simulink model "BaseEngineController_LS_128"  (Simulink 7.7)
settings: Solver=FixedStepDiscrete  StartTime=0.0  StopTime=10.0  RelTol=1e-3
PreLoadFcn:
  | try, eval([bdroot '_setup']); catch, eval('model_setup', ''); end
InitFcn:
  | try, eval([bdroot '_setup']); catch, eval('model_setup', ''); end
undefined symbols (not defined in the file): ECU565, High, motohawk_build_version, motohawk_trunc_name, motohawk_vardec_config_group, motohawk_vardec_path, True
libraries: MotoHawk_lib x1418, motohawk_control_primitives_lib x183, motohawk_engine_lib x32, simulink x21, motohawk_annotations_lib x9, AutoDoc_lib x8, simulink_extras x4, motohawk_ccp_examples_lib x1, motohawk_control_primitives_motoshare_lib x1
(part 25 of 27)

== system BaseEngineController_LS_128/Foreground/Control/Controller/Run/Fuel System Manager/O2 Fuel Adapt/Saturation (Tunable)1 ==
  note: Calibratable wrapper around the Saturation block
  In : Inport
  Saturation : motohawk_control_primitives_lib/Saturation  SystemSampleTime=-1
  motohawk_calibration : MotoHawk_lib/Calibration & Probing Blocks/motohawk_calibration  nam=[prefix 'LwrLim']  val=LwrLim  storage=Calibration  show_more=on  name_source=Use Parameter  data_type=Inherit via back propagation  read_level=1  write_level=1  ovr_cals=on  view_as=Number  enum_struct={'Disabled', 'Enabled'}  vector_style=Wide Row  use_help_units=off  help='Lower Limit Value'  units=units  use_header_enum=off  row_header_enum={}  col_header_enum={}  use_min_max=on  min_val=-inf  max_val=inf  use_precision=on  precision='1.4'  gain=1  offset=0  exp=1  use_mototune_group=on  mototune_group=motohawk_vardec_path(gcb)
  motohawk_calibration1 : MotoHawk_lib/Calibration & Probing Blocks/motohawk_calibration  nam=[prefix 'UprLim']  val=UprLim  storage=Calibration  show_more=on  name_source=Use Parameter  data_type=Inherit via back propagation  read_level=1  write_level=1  ovr_cals=on  view_as=Number  enum_struct={'Disabled', 'Enabled'}  vector_style=Wide Row  use_help_units=off  help='Upper Limit Value'  units=units  use_header_enum=off  row_header_enum={}  col_header_enum={}  use_min_max=on  min_val=-inf  max_val=inf  use_precision=on  precision='1.4'  gain=1  offset=0  exp=1  use_mototune_group=on  mototune_group=motohawk_vardec_path(gcb)
  Out : Outport
  wires:
  motohawk_calibration1/1 -> Saturation/3
  In/1 -> Saturation/1
  motohawk_calibration/1 -> Saturation/2
  Saturation/1 -> Out/1

== system BaseEngineController_LS_128/Foreground/Control/Controller/Run/Fuel System Manager/O2 Fuel Adapt/WarmUp Disable ==
  WarmupRatio : Inport
  WarmupTimeRatio : Inport  Port=2
  BaseRatio : Inport  Port=3
  Constant : Constant  Value=0.01
  Logical Operator : Logic  Operator=NOT  AllPortsSameDT=off
  MinMax : MinMax  Function=max  Inputs=2
  Relational Operator : RelationalOperator  Operator=>  InputSameDT=on
  Sum : Sum  Inputs=|+-
  motohawk_probe5 : MotoHawk_lib/Calibration & Probing Blocks/motohawk_probe  nam='WarmUpO2AdaptEnabled'  show_more=on  name_source=Use Parameter  read_level=1  view_as=Enumeration  enum_struct={'Not Enabled', 'Enabled'}  vector_style=Wide Row  use_help_units=on  help='Indicates whether FuelFlowComp map adapting is enabled due to WarmUp'  units=''  use_header_enum=off  row_header_enum={}  col_header_enum={}  use_precision=off  precision=''  gain=1  offset=0  exp=1  use_mototune_group=on  mototune_group=motohawk_vardec_path(gcb)
  State_Out : Outport
  wires:
  Relational Operator/1 -> Logical Operator/1
  Logical Operator/1 -> State_Out/1, motohawk_probe5/1
  Constant/1 -> Relational Operator/2
  WarmupRatio/1 -> MinMax/1
  WarmupTimeRatio/1 -> MinMax/2
  MinMax/1 -> Sum/1
  BaseRatio/1 -> Sum/2
  Sum/1 -> Relational Operator/1

== system BaseEngineController_LS_128/Foreground/Control/Controller/Run/MaxGovernor/Trigger Pre-load/InGear ==
  Enable : EnablePort
  Saturation : motohawk_control_primitives_lib/Saturation  SystemSampleTime=-1
  motohawk_calibration2 : MotoHawk_lib/Calibration & Probing Blocks/motohawk_calibration  nam='MaxGovInGearRPMSetPt'  val=4200  storage=Calibration  show_more=on  name_source=Use Parameter  data_type=uint16  read_level=1  write_level=1  ovr_cals=on  view_as=Number  enum_struct={'Disabled', 'Enabled'}  vector_style=Wide Row  use_help_units=on  help='Max Gov RPM setpoint when in gear.'  units='RPM'  use_header_enum=off  row_header_enum={}  col_header_enum={}  use_min_max=on  min_val=0  max_val=inf  use_precision=off  precision=''  gain=1  offset=0  exp=1  use_mototune_group=on  mototune_group=motohawk_vardec_path(gcb)
  motohawk_calibration3 : MotoHawk_lib/Calibration & Probing Blocks/motohawk_calibration  nam='MaxGovInGearLowerLim'  val=300  storage=Calibration  show_more=on  name_source=Use Parameter  data_type=uint16  read_level=1  write_level=1  ovr_cals=on  view_as=Number  enum_struct={'Disabled', 'Enabled'}  vector_style=Wide Row  use_help_units=on  help='Max Gov RPM setpoint when in gear.'  units='RPM'  use_header_enum=off  row_header_enum={}  col_header_enum={}  use_min_max=on  min_val=0  max_val=inf  use_precision=off  precision=''  gain=1  offset=0  exp=1  use_mototune_group=on  mototune_group=motohawk_vardec_path(gcb)
  motohawk_calibration4 : MotoHawk_lib/Calibration & Probing Blocks/motohawk_calibration  nam='MaxGovInGearRPMThresh'  val=300  storage=Calibration  show_more=on  name_source=Use Parameter  data_type=uint16  read_level=1  write_level=1  ovr_cals=on  view_as=Number  enum_struct={'Disabled', 'Enabled'}  vector_style=Wide Row  use_help_units=on  help='When in-gear, RPM has to pass the base RPM setpoint minus this calibration. to start the I term preload and ramp-in.'  units='RPM'  use_header_enum=off  row_header_enum={}  col_header_enum={}  use_min_max=off  min_val=0  max_val=inf  use_precision=off  precision=''  gain=1  offset=0  exp=1  use_mototune_group=on  mototune_group=motohawk_vardec_path(gcb)
  motohawk_calibration5 : MotoHawk_lib/Calibration & Probing Blocks/motohawk_calibration  nam='MaxGovInGearUpperLim'  val=4200  storage=Calibration  show_more=on  name_source=Use Parameter  data_type=uint16  read_level=1  write_level=1  ovr_cals=on  view_as=Number  enum_struct={'Disabled', 'Enabled'}  vector_style=Wide Row  use_help_units=on  help='Max Gov RPM setpoint when in gear.'  units='RPM'  use_header_enum=off  row_header_enum={}  col_header_enum={}  use_min_max=on  min_val=0  max_val=inf  use_precision=off  precision=''  gain=1  offset=0  exp=1  use_mototune_group=on  mototune_group=motohawk_vardec_path(gcb)
  motohawk_data_def : MotoHawk_lib/Data Storage Blocks/motohawk_data_def  nam='MaxGovInGearSetPoint'  container_nam=''  data=3500  typ=uint16  struct_nam='MyStruct'  storage=NonVolatile  outputRef=off  use_vardec=off  window=Calibration  read_level=1  write_level=1  ovr_cals=on  view_as=Number  enum_struct={'Disabled', 'Enabled'}  vector_style=Wide Row  use_help_units=on  help=''  units=''  use_header_enum=off  row_header_enum=''  col_header_enum=''  use_min_max=off  min_val=-inf  max_val=inf  use_precision=off  precision=''  gain=1  offset=0  exp=1  use_mototune_group=off  mototune_group=motohawk_vardec_path(gcb)  eval_name=MaxGovInGearSetPoint  data_stores=motohawk_sfun_data_def_data_stores  struct_instances=motohawk_sfun_data_def_struct_instances  vardecs=motohawk_sfun_data_def_vardecs
  motohawk_data_read : MotoHawk_lib/Data Storage Blocks/motohawk_data_read  source=Lookup By Name  structure=Scalar  operation=Read scalar from location by index  sz_vec=4  sz_row=2  sz_col=3  typ=uint16  nam='MaxGovInGearSetPoint'  checkNull=on  struct_inst_name='Struct1'  struct_nam='MyStruct'
  motohawk_data_write1 : MotoHawk_lib/Data Storage Blocks/motohawk_data_write  source=Lookup By Name  structure=Scalar  operation=Write scalar into location by index  sz_vec=-1  sz_row=3  sz_col=2  typ=uint16  nam='MaxGovInGearSetPoint'  checkNull=on  write_read_only=off  struct_inst_name='Struct1'  struct_name='MyStruct'
  BaseSetpoint : Outport
  Threshold : Outport  Port=2
  wires:
  motohawk_calibration4/1 -> Threshold/1
  motohawk_calibration2/1 -> motohawk_data_write1/1
  motohawk_data_read/1 -> Saturation/1
  Saturation/1 -> BaseSetpoint/1
  motohawk_calibration3/1 -> Saturation/2
  motohawk_calibration5/1 -> Saturation/3

== system BaseEngineController_LS_128/Foreground/Control/Controller/Run/MaxGovernor/Trigger Pre-load/InNeutral ==
  Enable : EnablePort
  Saturation : motohawk_control_primitives_lib/Saturation  SystemSampleTime=-1
  motohawk_calibration2 : MotoHawk_lib/Calibration & Probing Blocks/motohawk_calibration  nam='MaxGovNtrlLowerLim'  val=2000  storage=Calibration  show_more=on  name_source=Use Parameter  data_type=uint16  read_level=1  write_level=1  ovr_cals=on  view_as=Number  enum_struct={'Disabled', 'Enabled'}  vector_style=Wide Row  use_help_units=on  help='Max Gov RPM setpoint when in gear.'  units='RPM'  use_header_enum=off  row_header_enum={}  col_header_enum={}  use_min_max=on  min_val=0  max_val=inf  use_precision=off  precision=''  gain=1  offset=0  exp=1  use_mototune_group=on  mototune_group=motohawk_vardec_path(gcb)
  motohawk_calibration3 : MotoHawk_lib/Calibration & Probing Blocks/motohawk_calibration  nam='MaxGovNtrlRPMThresh'  val=300  storage=Calibration  show_more=on  name_source=Use Parameter  data_type=uint16  read_level=1  write_level=1  ovr_cals=on  view_as=Number  enum_struct={'Disabled', 'Enabled'}  vector_style=Wide Row  use_help_units=on  help='When in neutral, RPM has to pass the base RPM setpoint minus this calibration. to start the I term preload and ramp-in.'  units='RPM'  use_header_enum=off  row_header_enum={}  col_header_enum={}  use_min_max=off  min_val=0  max_val=inf  use_precision=off  precision=''  gain=1  offset=0  exp=1  use_mototune_group=on  mototune_group=motohawk_vardec_path(gcb)
  motohawk_calibration4 : MotoHawk_lib/Calibration & Probing Blocks/motohawk_calibration  nam='MaxGovNtrlRPMSetPt'  val=3500  storage=Calibration  show_more=on  name_source=Use Parameter  data_type=uint16  read_level=1  write_level=1  ovr_cals=on  view_as=Number  enum_struct={'Disabled', 'Enabled'}  vector_style=Wide Row  use_help_units=on  help='Max Gov RPM setpoint when in neutral.'  units='RPM'  use_header_enum=off  row_header_enum={}  col_header_enum={}  use_min_max=on  min_val=0  max_val=inf  use_precision=off  precision=''  gain=1  offset=0  exp=1  use_mototune_group=on  mototune_group=motohawk_vardec_path(gcb)
  motohawk_calibration5 : MotoHawk_lib/Calibration & Probing Blocks/motohawk_calibration  nam='MaxGovNtrlUpperLim'  val=4000  storage=Calibration  show_more=on  name_source=Use Parameter  data_type=uint16  read_level=1  write_level=1  ovr_cals=on  view_as=Number  enum_struct={'Disabled', 'Enabled'}  vector_style=Wide Row  use_help_units=on  help='Max Gov RPM setpoint when in gear.'  units='RPM'  use_header_enum=off  row_header_enum={}  col_header_enum={}  use_min_max=on  min_val=0  max_val=inf  use_precision=off  precision=''  gain=1  offset=0  exp=1  use_mototune_group=on  mototune_group=motohawk_vardec_path(gcb)
  motohawk_data_def : MotoHawk_lib/Data Storage Blocks/motohawk_data_def  nam='MaxGovNtrlSetPoint'  container_nam=''  data=3500  typ=uint16  struct_nam='MyStruct'  storage=NonVolatile  outputRef=off  use_vardec=off  window=Calibration  read_level=1  write_level=1  ovr_cals=on  view_as=Number  enum_struct={'Disabled', 'Enabled'}  vector_style=Wide Row  use_help_units=on  help=''  units=''  use_header_enum=off  row_header_enum=''  col_header_enum=''  use_min_max=off  min_val=-inf  max_val=inf  use_precision=off  precision=''  gain=1  offset=0  exp=1  use_mototune_group=off  mototune_group=motohawk_vardec_path(gcb)  eval_name=MaxGovNtrlSetPoint  data_stores=motohawk_sfun_data_def_data_stores  struct_instances=motohawk_sfun_data_def_struct_instances  vardecs=motohawk_sfun_data_def_vardecs
  motohawk_data_read : MotoHawk_lib/Data Storage Blocks/motohawk_data_read  source=Lookup By Name  structure=Scalar  operation=Read scalar from location by index  sz_vec=4  sz_row=2  sz_col=3  typ=uint16  nam='MaxGovNtrlSetPoint'  checkNull=on  struct_inst_name='Struct1'  struct_nam='MyStruct'
  motohawk_data_write1 : MotoHawk_lib/Data Storage Blocks/motohawk_data_write  source=Lookup By Name  structure=Scalar  operation=Write scalar into location by index  sz_vec=-1  sz_row=3  sz_col=2  typ=uint16  nam='MaxGovNtrlSetPoint'  checkNull=on  write_read_only=off  struct_inst_name='Struct1'  struct_name='MyStruct'
  BaseSetpoint : Outport
  Threshold : Outport  Port=2
  wires:
  motohawk_calibration3/1 -> Threshold/1
  motohawk_calibration4/1 -> motohawk_data_write1/1
  motohawk_data_read/1 -> Saturation/1
  motohawk_calibration2/1 -> Saturation/2
  motohawk_calibration5/1 -> Saturation/3
  Saturation/1 -> BaseSetpoint/1

== system BaseEngineController_LS_128/Foreground/Control/Controller/Run/MinGovernor/AiflowOffset/Ramp Air Into Idle State ==
  note: 1st-Order Ramp Down
  note: y[k] = a*x[k] + (1-a)*y[k-1]
  note: where a = t/T
  EngineState : Inport
  TPSOffset : Inport  Port=2
  InitialSetpoint : Inport  Port=3
  Constant : Constant  OutDataTypeStr=Inherit: Inherit via back propagation
  Don't allow setpoint to ever drop below the TargetRPM : MinMax  Function=max  Inputs=2  SaturateOnIntegerOverflow=on  InputSameDT=on
  Logical Operator : Logic  Operator=NOT
  Preload lowpass filter with current RPM while not on Idle : Switch  Threshold=0.5  ZeroCross=off  SaturateOnIntegerOverflow=on  InputSameDT=on
  Product1 : Product  Inputs=*/  SaturateOnIntegerOverflow=on  InputSameDT=on  OutDataTypeStr=Inherit: Same as first input
  Product2 : Product  SaturateOnIntegerOverflow=on  InputSameDT=on  OutDataTypeStr=Inherit: Same as first input
  Product3 : Product  SaturateOnIntegerOverflow=on  InputSameDT=on  OutDataTypeStr=Inherit: Same as first input
  Sum : Sum  Inputs=-+|  SaturateOnIntegerOverflow=on
  Sum1 : Sum  SaturateOnIntegerOverflow=on
  Unit Delay : UnitDelay  SampleTime=-1
  motohawk_calibration2 : MotoHawk_lib/Calibration & Probing Blocks/motohawk_calibration  nam='IdleEntryAirRampInFiltC'  val=0.1  storage=Calibration  show_more=on  name_source=Use Parameter  data_type=Inherit from 'Default Value'  read_level=1  write_level=1  ovr_cals=on  view_as=Number  enum_struct={'Disabled', 'Enabled'}  vector_style=Wide Row  use_help_units=on  help='Decays TPS Setpoint from Crank TPS to Run State base value at this rate.'  units='sec'  use_header_enum=off  row_header_enum={}  col_header_enum={}  use_min_max=on  min_val=.005  max_val=inf  use_precision=off  precision=''  gain=1  offset=0  exp=1  use_mototune_group=on  mototune_group=motohawk_vardec_path(gcb)
  motohawk_delta_time : MotoHawk_lib/Extra Development Blocks/motohawk_delta_time  samp_time=-1  init_val=0  mode=Seconds (double)
  TPSSetpoint : Outport
  wires:
  Logical Operator/1 -> Preload lowpass filter with current RPM while not on Idle/2
  Don't allow setpoint to ever drop below the TargetRPM/1 -> TPSSetpoint/1, Unit Delay/1
  Preload lowpass filter with current RPM while not on Idle/1 -> Don't allow setpoint to ever drop below the TargetRPM/2
  InitialSetpoint/1 -> Preload lowpass filter with current RPM while not on Idle/1
  TPSOffset/1 -> Don't allow setpoint to ever drop below the TargetRPM/1, Product2/1
  Product1/1 -> Sum/1, Product2/2  "alpha"
  Constant/1 -> Sum/2
  Product2/1 -> Sum1/1
  Product3/1 -> Sum1/2
  Sum/1 -> Product3/1
  Unit Delay/1 -> Product3/2
  motohawk_delta_time/1 -> Product1/1
  motohawk_calibration2/1 -> Product1/2
  Sum1/1 -> Preload lowpass filter with current RPM while not on Idle/3
  EngineState/1 -> Logical Operator/1

== system BaseEngineController_LS_128/Foreground/Control/Controller/Run/MinGovernor/Base Airflow Table Adapt/Adapt Base Airflow Table ==
  error : Inport
  Enable : EnablePort
  motohawk_adapt_table : MotoHawk_lib/Lookup Tables/motohawk_adapt_table  nam='BaseAirflowOfstTbl'  typ=double  mode=Adapt between points  show_adapted=off
  motohawk_calibration1 : MotoHawk_lib/Calibration & Probing Blocks/motohawk_calibration  nam='BaseAirflowOfstMinValue'  val=0  storage=Calibration  show_more=on  name_source=Use Parameter  data_type=Inherit from 'Default Value'  read_level=1  write_level=1  ovr_cals=on  view_as=Number  enum_struct={'Disabled', 'Enabled'}  vector_style=Wide Row  use_help_units=on  help='Minimum value that can be adapted into the BaseAirflowOfst table.'  units='%'  use_header_enum=off  row_header_enum={}  col_header_enum={}  use_min_max=on  min_val=-inf  max_val=inf  use_precision=off  precision=''  gain=1  offset=0  exp=1  use_mototune_group=on  mototune_group=motohawk_vardec_path(gcb)
  motohawk_calibration2 : MotoHawk_lib/Calibration & Probing Blocks/motohawk_calibration  nam='BaseAirflowOfstMaxValue'  val=0  storage=Calibration  show_more=on  name_source=Use Parameter  data_type=Inherit from 'Default Value'  read_level=1  write_level=1  ovr_cals=on  view_as=Number  enum_struct={'Disabled', 'Enabled'}  vector_style=Wide Row  use_help_units=on  help='Maximum value that can be adapted into the BaseAirflowOfst table.'  units='%'  use_header_enum=off  row_header_enum={}  col_header_enum={}  use_min_max=on  min_val=-inf  max_val=inf  use_precision=off  precision=''  gain=1  offset=0  exp=1  use_mototune_group=on  mototune_group=motohawk_vardec_path(gcb)
  wires:
  error/1 -> motohawk_adapt_table/1
  motohawk_calibration1/1 -> motohawk_adapt_table/2
  motohawk_calibration2/1 -> motohawk_adapt_table/3

== system BaseEngineController_LS_128/Foreground/Control/Controller/Run/MinGovernor/Base Airflow Table Adapt/Idle Control Enable Delay ==
  State_In : Inport
  Relational Operator : RelationalOperator  Operator=>  InputSameDT=on
  Time Since Enabled (With Input)1 : motohawk_control_primitives_lib/Time Since Enabled (With Input)1  SystemSampleTime=-1  nam='BaseAirflowTimer'  samp_time=.005  init=0  upperlim=16000
  motohawk_calibration1 : MotoHawk_lib/Calibration & Probing Blocks/motohawk_calibration  nam='BaseAirflowAdaptDelayTime'  val=5  storage=Calibration  show_more=on  name_source=Use Parameter  data_type=Inherit from 'Default Value'  read_level=1  write_level=1  ovr_cals=on  view_as=Number  enum_struct={'Disabled', 'Enabled'}  vector_style=Wide Row  use_help_units=on  help='Idle Control must be enabled for this amount of time before fuel adaption is enabled'  units='s'  use_header_enum=off  row_header_enum={}  col_header_enum={}  use_min_max=off  min_val=0  max_val=inf  use_precision=off  precision=''  gain=1  offset=0  exp=1  use_mototune_group=on  mototune_group=motohawk_vardec_path(gcb)
  State_Out : Outport
  wires:
  State_In/1 -> Time Since Enabled (With Input)1/1
  motohawk_calibration1/1 -> Relational Operator/2
  Time Since Enabled (With Input)1/1 -> Relational Operator/1
  Relational Operator/1 -> State_Out/1

== system BaseEngineController_LS_128/Foreground/Control/Controller/Run/MinGovernor/Base Airflow Table Adapt/Saturation (Tunable) ==
  note: Calibratable wrapper around the Saturation block
  In : Inport
  Saturation : motohawk_control_primitives_lib/Saturation  SystemSampleTime=-1
  motohawk_calibration : MotoHawk_lib/Calibration & Probing Blocks/motohawk_calibration  nam=[prefix 'LwrLim']  val=LwrLim  storage=Calibration  show_more=on  name_source=Use Parameter  data_type=Inherit via back propagation  read_level=1  write_level=1  ovr_cals=on  view_as=Number  enum_struct={'Disabled', 'Enabled'}  vector_style=Wide Row  use_help_units=off  help='Lower Limit Value'  units=units  use_header_enum=off  row_header_enum={}  col_header_enum={}  use_min_max=on  min_val=-inf  max_val=inf  use_precision=on  precision='1.4'  gain=1  offset=0  exp=1  use_mototune_group=on  mototune_group=motohawk_vardec_path(gcb)
  motohawk_calibration1 : MotoHawk_lib/Calibration & Probing Blocks/motohawk_calibration  nam=[prefix 'UprLim']  val=UprLim  storage=Calibration  show_more=on  name_source=Use Parameter  data_type=Inherit via back propagation  read_level=1  write_level=1  ovr_cals=on  view_as=Number  enum_struct={'Disabled', 'Enabled'}  vector_style=Wide Row  use_help_units=off  help='Upper Limit Value'  units=units  use_header_enum=off  row_header_enum={}  col_header_enum={}  use_min_max=on  min_val=-inf  max_val=inf  use_precision=on  precision='1.4'  gain=1  offset=0  exp=1  use_mototune_group=on  mototune_group=motohawk_vardec_path(gcb)
  Out : Outport
  wires:
  motohawk_calibration1/1 -> Saturation/3
  In/1 -> Saturation/1
  motohawk_calibration/1 -> Saturation/2
  Saturation/1 -> Out/1

== system BaseEngineController_LS_128/Foreground/Control/Controller/Run/MinGovernor/Idle State Determination/Determine if RPM is Falling ==
  note: Determine if RPM is falling
  RPM : Inport
  Derivitive : motohawk_control_primitives_lib/Derivitive  SystemSampleTime=-1  samp_time=.005
  Falling RPM is Negative Derivative : Gain  Gain=-1  OutDataTypeStr=Inherit: Same as input  ParamDataTypeStr=Inherit: Same as input
  First Order Low Pass (Tunable) : motohawk_control_primitives_lib/First Order Low Pass (Tunable)  SystemSampleTime=-1  nam='RPMFallingFiltConst'  samp_time=.005  group=motohawk_vardec_path(gcb)
  Relational Operator : RelationalOperator  Operator=<
  motohawk_calibration : MotoHawk_lib/Calibration & Probing Blocks/motohawk_calibration  nam='RPMFallingRate'  val=0.05  storage=Calibration  show_more=on  name_source=Use Parameter  data_type=Inherit from 'Default Value'  read_level=1  write_level=1  ovr_cals=on  view_as=Number  enum_struct={'Disabled', 'Enabled'}  vector_style=Wide Row  use_help_units=on  help='The minimum rate of change in RPM that triggers RPMFalling - This should be a positive value'  units='RPM/sec'  use_header_enum=off  row_header_enum={}  col_header_enum={}  use_min_max=on  min_val=0  max_val=1000  use_precision=off  precision=''  gain=1  offset=0  exp=1  use_mototune_group=on  mototune_group=motohawk_vardec_path(gcb)
  motohawk_probe : MotoHawk_lib/Calibration & Probing Blocks/motohawk_probe  nam='RPMFalling'  show_more=on  name_source=Use Parameter  read_level=1  view_as=Enumeration  enum_struct={'SteadyOrRising', 'Falling'}  vector_style=Wide Row  use_help_units=on  help='Indicates whether the RPM is falling'  units=''  use_header_enum=off  row_header_enum={}  col_header_enum={}  use_precision=off  precision=''  gain=1  offset=0  exp=1  use_mototune_group=on  mototune_group=motohawk_vardec_path(gcb)
  RPM Falling : Outport
  wires:
  Falling RPM is Negative Derivative/1 -> Relational Operator/2
  RPM/1 -> Derivitive/1
  Relational Operator/1 -> RPM Falling/1, motohawk_probe/1
  motohawk_calibration/1 -> Falling RPM is Negative Derivative/1
  First Order Low Pass (Tunable)/1 -> Relational Operator/1
  Derivitive/1 -> First Order Low Pass (Tunable)/1

== system BaseEngineController_LS_128/Foreground/Control/Controller/Run/MinGovernor/Universal PD (Tunable & Scheduled)/PID Gain Select ==
  ErrorIdx : Inport
  Product1 : Product  SaturateOnIntegerOverflow=on  InputSameDT=on  OutDataTypeStr=Inherit: Same as first input
  Product2 : Product  SaturateOnIntegerOverflow=on  InputSameDT=on  OutDataTypeStr=Inherit: Same as first input
  motohawk_calibration1 : MotoHawk_lib/Calibration & Probing Blocks/motohawk_calibration  nam=[prefix 'DGain']  val=0  storage=Calibration  show_more=on  name_source=Use Parameter  data_type=Inherit from 'Default Value'  read_level=1  write_level=1  ovr_cals=on  view_as=Number  enum_struct={'Disabled', 'Enabled'}  vector_style=Wide Row  use_help_units=on  help='Base D-gain for the min. governor controller.'  units='mult'  use_header_enum=off  row_header_enum={}  col_header_enum={}  use_min_max=off  min_val=-inf  max_val=inf  use_precision=off  precision=''  gain=1  offset=0  exp=1  use_mototune_group=on  mototune_group=motohawk_vardec_path(gcb)
  motohawk_calibration3 : MotoHawk_lib/Calibration & Probing Blocks/motohawk_calibration  nam=[prefix 'PGain']  val=0  storage=Calibration  show_more=on  name_source=Use Parameter  data_type=Inherit from 'Default Value'  read_level=1  write_level=1  ovr_cals=on  view_as=Number  enum_struct={'Disabled', 'Enabled'}  vector_style=Wide Row  use_help_units=on  help='Base P-gain for the min. governor controller.'  units='mult'  use_header_enum=off  row_header_enum={}  col_header_enum={}  use_min_max=off  min_val=-inf  max_val=inf  use_precision=off  precision=''  gain=1  offset=0  exp=1  use_mototune_group=on  mototune_group=motohawk_vardec_path(gcb)
  motohawk_interpolation_1d1 : MotoHawk_lib/Lookup Tables/motohawk_interpolation_1d  nam=[prefix 'DGainErrorMult']  table_data=[0.5 0.3 0.01 0.01 0.2 0.5 1 1.3 1.5]  show_more=on  data_type=Inherit from 'Table Data'  storage=NonAdaptive  read_level=1  write_level=1  ovr_cals=on  use_help=on  help=''  units='mult'  use_min_max=on  min_val=-inf  max_val=inf  use_precision=off  precision=''  gain=1  offset=0  exp=1  use_links=off  prelookup_block=''  output_name=''  use_mototune_group=on  mototune_group=motohawk_vardec_path(gcb)
  motohawk_interpolation_1d2 : MotoHawk_lib/Lookup Tables/motohawk_interpolation_1d  nam=[prefix 'PGainErrorMult']  table_data=[0.5 0.3 0.01 0.01 0.2 0.5 1 1.3 1.5]  show_more=on  data_type=Inherit from 'Table Data'  storage=NonAdaptive  read_level=1  write_level=1  ovr_cals=on  use_help=on  help=''  units='mult'  use_min_max=on  min_val=-inf  max_val=inf  use_precision=off  precision=''  gain=1  offset=0  exp=1  use_links=off  prelookup_block=''  output_name=''  use_mototune_group=on  mototune_group=motohawk_vardec_path(gcb)
  PGain : Outport
  DGain : Outport  Port=2
  wires:
  motohawk_calibration3/1 -> Product2/1
  Product2/1 -> PGain/1
  motohawk_interpolation_1d2/1 -> Product2/2
  ErrorIdx/1 -> motohawk_interpolation_1d2/1, motohawk_interpolation_1d1/1
  motohawk_calibration1/1 -> Product1/1
  Product1/1 -> DGain/1
  motohawk_interpolation_1d1/1 -> Product1/2

== system BaseEngineController_LS_128/Foreground/Control/Controller/Run/MinGovernor/Universal PID (Tunable & Scheduled)/PID Gain Select1 ==
  ErrorIdx : Inport
  Product1 : Product  SaturateOnIntegerOverflow=on  InputSameDT=on  OutDataTypeStr=Inherit: Same as first input
  Product2 : Product  SaturateOnIntegerOverflow=on  InputSameDT=on  OutDataTypeStr=Inherit: Same as first input
  Product3 : Product  SaturateOnIntegerOverflow=on  InputSameDT=on  OutDataTypeStr=Inherit: Same as first input
  motohawk_calibration1 : MotoHawk_lib/Calibration & Probing Blocks/motohawk_calibration  nam=[prefix 'IGain']  val=0  storage=Calibration  show_more=on  name_source=Use Parameter  data_type=Inherit from 'Default Value'  read_level=1  write_level=1  ovr_cals=on  view_as=Number  enum_struct={'Disabled', 'Enabled'}  vector_style=Wide Row  use_help_units=on  help='Base I-gain for the min. governor controller.'  units='mult'  use_header_enum=off  row_header_enum={}  col_header_enum={}  use_min_max=off  min_val=-inf  max_val=inf  use_precision=off  precision=''  gain=1  offset=0  exp=1  use_mototune_group=on  mototune_group=motohawk_vardec_path(gcb)
  motohawk_calibration2 : MotoHawk_lib/Calibration & Probing Blocks/motohawk_calibration  nam=[prefix 'DGain']  val=0  storage=Calibration  show_more=on  name_source=Use Parameter  data_type=Inherit from 'Default Value'  read_level=1  write_level=1  ovr_cals=on  view_as=Number  enum_struct={'Disabled', 'Enabled'}  vector_style=Wide Row  use_help_units=on  help='Base D-gain for the min. governor controller.'  units='mult'  use_header_enum=off  row_header_enum={}  col_header_enum={}  use_min_max=off  min_val=-inf  max_val=inf  use_precision=off  precision=''  gain=1  offset=0  exp=1  use_mototune_group=on  mototune_group=motohawk_vardec_path(gcb)
  motohawk_calibration3 : MotoHawk_lib/Calibration & Probing Blocks/motohawk_calibration  nam=[prefix 'PGain']  val=0  storage=Calibration  show_more=on  name_source=Use Parameter  data_type=Inherit from 'Default Value'  read_level=1  write_level=1  ovr_cals=on  view_as=Number  enum_struct={'Disabled', 'Enabled'}  vector_style=Wide Row  use_help_units=on  help='Base P-gain for the min. governor controller.'  units='mult'  use_header_enum=off  row_header_enum={}  col_header_enum={}  use_min_max=off  min_val=-inf  max_val=inf  use_precision=off  precision=''  gain=1  offset=0  exp=1  use_mototune_group=on  mototune_group=motohawk_vardec_path(gcb)
  motohawk_interpolation_1d1 : MotoHawk_lib/Lookup Tables/motohawk_interpolation_1d  nam=[prefix 'IGainErrorMult']  table_data=[0.5 0.3 0.01 0.01 0.2 0.5 1 1.3 1.5]  show_more=on  data_type=Inherit from 'Table Data'  storage=NonAdaptive  read_level=1  write_level=1  ovr_cals=on  use_help=on  help=''  units='mult'  use_min_max=on  min_val=-inf  max_val=inf  use_precision=off  precision=''  gain=1  offset=0  exp=1  use_links=off  prelookup_block=''  output_name=''  use_mototune_group=on  mototune_group=motohawk_vardec_path(gcb)
  motohawk_interpolation_1d2 : MotoHawk_lib/Lookup Tables/motohawk_interpolation_1d  nam=[prefix 'PGainErrorMult']  table_data=[0.5 0.3 0.01 0.01 0.2 0.5 1 1.3 1.5]  show_more=on  data_type=Inherit from 'Table Data'  storage=NonAdaptive  read_level=1  write_level=1  ovr_cals=on  use_help=on  help=''  units='mult'  use_min_max=on  min_val=-inf  max_val=inf  use_precision=off  precision=''  gain=1  offset=0  exp=1  use_links=off  prelookup_block=''  output_name=''  use_mototune_group=on  mototune_group=motohawk_vardec_path(gcb)
  motohawk_interpolation_1d3 : MotoHawk_lib/Lookup Tables/motohawk_interpolation_1d  nam=[prefix 'DGainErrorMult']  table_data=[0.5 0.3 0.01 0.01 0.2 0.5 1 1.3 1.5]  show_more=on  data_type=Inherit from 'Table Data'  storage=NonAdaptive  read_level=1  write_level=1  ovr_cals=on  use_help=on  help=''  units='mult'  use_min_max=on  min_val=-inf  max_val=inf  use_precision=off  precision=''  gain=1  offset=0  exp=1  use_links=off  prelookup_block=''  output_name=''  use_mototune_group=on  mototune_group=motohawk_vardec_path(gcb)
  PGain : Outport
  IGain : Outport  Port=2
  DGain : Outport  Port=3
  wires:
  ErrorIdx/1 -> motohawk_interpolation_1d2/1, motohawk_interpolation_1d1/1, motohawk_interpolation_1d3/1
  motohawk_interpolation_1d2/1 -> Product2/2
  Product2/1 -> PGain/1
  motohawk_calibration3/1 -> Product2/1
  motohawk_calibration1/1 -> Product1/1
  motohawk_interpolation_1d1/1 -> Product1/2
  Product1/1 -> IGain/1
  motohawk_interpolation_1d3/1 -> Product3/2
  Product3/1 -> DGain/1
  motohawk_calibration2/1 -> Product3/1

== system BaseEngineController_LS_128/Foreground/Control/Controller/Run/O2 Control/O2 PID Calibrations/Error Gain Scheduling ==
  Sensors : Inport
  Bus Selector : BusSelector  OutputSignals=RawIndexes.ECT09Idx,VirtualIndexes.MAFPort05Idx
  Product : Product  RndMeth=Zero
  motohawk_interpolation_1d : MotoHawk_lib/Lookup Tables/motohawk_interpolation_1d  nam='O2NECCTErrGainMult'  table_data=[1 1 1 1 1 1 1 1 1]  show_more=on  data_type=Inherit from 'Table Data'  storage=NonAdaptive  read_level=1  write_level=1  ovr_cals=on  use_help=on  help='O2 PID controller system gain based on NECCT.'  units='mult'  use_min_max=off  min_val=-inf  max_val=inf  use_precision=on  precision='1.4'  gain=1  offset=0  exp=1  use_links=off  prelookup_block=''  output_name=''  use_mototune_group=on  mototune_group=motohawk_vardec_path(gcb)
  motohawk_interpolation_1d1 : MotoHawk_lib/Lookup Tables/motohawk_interpolation_1d  nam='O2MAFErrGainMult'  table_data=[0.1 0.1 0.3 0.5 0.6]  show_more=on  data_type=Inherit from 'Table Data'  storage=NonAdaptive  read_level=1  write_level=1  ovr_cals=on  use_help=on  help='O2 PID controller system gain based on MAF port.'  units='mult'  use_min_max=off  min_val=-inf  max_val=inf  use_precision=on  precision='1.4'  gain=1  offset=0  exp=1  use_links=off  prelookup_block=''  output_name=''  use_mototune_group=on  mototune_group=motohawk_vardec_path(gcb)
  ErrorGain : Outport
  wires:
  Bus Selector/1 -> motohawk_interpolation_1d/1  "<ECT09Idx>"
  Sensors/1 -> Bus Selector/1
  Product/1 -> ErrorGain/1
  motohawk_interpolation_1d/1 -> Product/1
  Bus Selector/2 -> motohawk_interpolation_1d1/1  "<MAFPort05Idx>"
  motohawk_interpolation_1d1/1 -> Product/2

== system BaseEngineController_LS_128/Foreground/Control/Controller/Run/O2 Control/O2 PID Calibrations/O2 Control Switch Point Maps ==
  Sensors : Inport
  Bus Selector : BusSelector  OutputSignals=RawIndexes.MAP09Idx,RawIndexes.RPM09Idx
  Documentation_Left_Border : AutoDoc_lib/Documentation_Left_Border  layout=Portrait
  motohawk_interpolation_2d : MotoHawk_lib/Lookup Tables/motohawk_interpolation_2d  nam='RichTargetDelta'  table_data=ones(9)  show_more=on  data_type=Inherit from 'Table Data'  storage=NonAdaptive  read_level=1  write_level=1  ovr_cals=on  use_help=on  help='Target on the rich side for perturbation.'  units='EquivRatio'  use_min_max=off  min_val=-inf  max_val=inf  use_precision=on  precision=''  gain=1  offset=0  exp=1  use_links=off  row_prelookup_block=''  col_prelookup_block=''  output_name=''  use_mototune_group=on  mototune_group=motohawk_vardec_path(gcb)
  motohawk_interpolation_2d1 : MotoHawk_lib/Lookup Tables/motohawk_interpolation_2d  nam='LeanTargetDelta'  table_data=ones(9)  show_more=on  data_type=Inherit from 'Table Data'  storage=NonAdaptive  read_level=1  write_level=1  ovr_cals=on  use_help=on  help='Target on the lean side for perturbation.'  units='EquivRatio'  use_min_max=off  min_val=-inf  max_val=inf  use_precision=on  precision=''  gain=1  offset=0  exp=1  use_links=off  row_prelookup_block=''  col_prelookup_block=''  output_name=''  use_mototune_group=on  mototune_group=motohawk_vardec_path(gcb)
  motohawk_interpolation_2d2 : MotoHawk_lib/Lookup Tables/motohawk_interpolation_2d  nam='RichSwPtDelta'  table_data=ones(9)  show_more=on  data_type=Inherit from 'Table Data'  storage=NonAdaptive  read_level=1  write_level=1  ovr_cals=on  use_help=on  help='If actual O2 reaches this point, switch the target to the LeanTargetDelta'  units='EquivRatio'  use_min_max=off  min_val=-inf  max_val=inf  use_precision=on  precision=''  gain=1  offset=0  exp=1  use_links=off  row_prelookup_block=''  col_prelookup_block=''  output_name=''  use_mototune_group=on  mototune_group=motohawk_vardec_path(gcb)
  motohawk_interpolation_2d3 : MotoHawk_lib/Lookup Tables/motohawk_interpolation_2d  nam='LeanSwPtDelta'  table_data=ones(9)  show_more=on  data_type=Inherit from 'Table Data'  storage=NonAdaptive  read_level=1  write_level=1  ovr_cals=on  use_help=on  help='If actual O2 reaches this point, switch the target to the RichTargetDelta'  units='EquivRatio'  use_min_max=off  min_val=-inf  max_val=inf  use_precision=on  precision=''  gain=1  offset=0  exp=1  use_links=off  row_prelookup_block=''  col_prelookup_block=''  output_name=''  use_mototune_group=on  mototune_group=motohawk_vardec_path(gcb)
  RichTargetDelta : Outport
  LeanTargetDelta : Outport  Port=2
  RichSwPtDelta : Outport  Port=3
  LeanSwPtDelta : Outport  Port=4
  wires:
  motohawk_interpolation_2d/1 -> RichTargetDelta/1  "RichEquivRatioTargetDelta"
  motohawk_interpolation_2d1/1 -> LeanTargetDelta/1  "LeanEquivRatioTargetDelta"
  motohawk_interpolation_2d2/1 -> RichSwPtDelta/1  "RichEquivRatioSwPtDelta"
  motohawk_interpolation_2d3/1 -> LeanSwPtDelta/1  "LeanEquivRatioSwPtDelta"
  Sensors/1 -> Bus Selector/1
  Bus Selector/1 -> motohawk_interpolation_2d3/1, motohawk_interpolation_2d2/1, motohawk_interpolation_2d1/1, motohawk_interpolation_2d/1  "<MAP09Idx>"
  Bus Selector/2 -> motohawk_interpolation_2d3/2, motohawk_interpolation_2d2/2, motohawk_interpolation_2d1/2, motohawk_interpolation_2d/2  "<RPM09Idx>"

== system BaseEngineController_LS_128/Foreground/Control/Controller/Run/O2 Control/O2 PID Controller Bank A/Closed-Loop O2 PID Controller ==
  O2Sensor : Inport
  TargetEquivRatio : Inport  Port=2
  ErrorGain : Inport  Port=3
  PGain : Inport  Port=4
  IGain : Inport  Port=5
  DGain : Inport  Port=6
  ITermUpperLimit : Inport  Port=7
  ITermLowerLimit : Inport  Port=8
  OutUpperLimit : Inport  Port=9
  OutLowerLimit : Inport  Port=10
  Reset : Inport  Port=11
  Constant : Constant  Value=0  OutDataTypeStr=Inherit: Inherit via back propagation
  Convert to Fuel Multiplier : Constant  OutDataTypeStr=Inherit: Inherit via back propagation
  Saturation : motohawk_control_primitives_lib/Saturation  SystemSampleTime=-1
  Sum : Sum  Inputs=++|  SaturateOnIntegerOverflow=on  InputSameDT=on
  Universal PID : motohawk_control_primitives_lib/Universal PID  Description=|  SystemSampleTime=-1  samp_time=.005
      | /* Name: ErrorGain Unit:mult ClassID:VAR StorageID:FLASH Access:RW4+RW3+NA2+NA1 TypeID:UINT4                   
      |    Gain:0.000000001 Min:0.000000000 Max:4.000000000 Format:10.9 UpdateID:REMOTE Help:"This gain is applied to "
      |    "the error term before it is used to calculate the P, I and D terms." VardecSig:6C */                       
      |                                                                                                                
      | /* Name: ITermLowerLim Unit:0 ClassID:VAR StorageID:FLASH Access:RW4+RW3+NA2+NA1 TypeID:SINT2 Gain:0.1         
      |    Min:-3276.8 Max:3276.7 Format:5.1 UpdateID:REMOTE Help:"Lower limit on the I-term value." VardecSig:6C */   
      |                                                                                                                
      | /* Name: ITermUpperLim ClassID:VAR StorageID:FLASH Access:RW4+RW3+NA2+NA1 TypeID:SINT2 Gain:0.1 Min:-3276.8    
      |    Max:3276.7 Format:5.1 UpdateID:REMOTE Help:"Upper limit on I-term value." VardecSig:6C */                   
      |                                                                                                                
      | /* Name: PIDOutLowerLim ClassID:VAR StorageID:FLASH Access:RW4+RW3+NA2+NA1 TypeID:SINT2 Gain:0.1               
      |    Min:-3276.8 Max:3276.7 Format:5.1 UpdateID:REMOTE Help:"Lower limit on PID output." VardecSig:6C */         
      |                                                                                                                
      | /* Name: PIDOutUpperLim ClassID:VAR StorageID:FLASH Access:RW4+RW3+NA2+NA1 TypeID:SINT2 Gain:0.1               
      |    Min:-3276.8 Max:3276.7 Format:3.1 UpdateID:REMOTE Help:"Upper limit on PID output." VardecSig:6C */
  motohawk_probe : MotoHawk_lib/Calibration & Probing Blocks/motohawk_probe  nam='LiquidO2Control_PTerm_BankA'  show_more=on  name_source=Use Parameter  read_level=1  view_as=Number  enum_struct={'Disabled', 'Enabled'}  vector_style=Wide Row  use_help_units=on  help='Closed-loop O2 control P-Term'  units='mult'  use_header_enum=off  row_header_enum={}  col_header_enum={}  use_precision=off  precision=''  gain=1  offset=0  exp=1  use_mototune_group=on  mototune_group=motohawk_vardec_path(gcb)
  motohawk_probe1 : MotoHawk_lib/Calibration & Probing Blocks/motohawk_probe  nam='LiquidO2Control_ITerm_BankA'  show_more=on  name_source=Use Parameter  read_level=1  view_as=Number  enum_struct={'Disabled', 'Enabled'}  vector_style=Wide Row  use_help_units=on  help='Closed-loop O2 control I-Term'  units='mult'  use_header_enum=off  row_header_enum={}  col_header_enum={}  use_precision=off  precision=''  gain=1  offset=0  exp=1  use_mototune_group=on  mototune_group=motohawk_vardec_path(gcb)
  motohawk_probe2 : MotoHawk_lib/Calibration & Probing Blocks/motohawk_probe  nam='LiquidO2Control_DTerm_BankA'  show_more=on  name_source=Use Parameter  read_level=1  view_as=Number  enum_struct={'Disabled', 'Enabled'}  vector_style=Wide Row  use_help_units=on  help='Closed-loop O2 control D-Term, for bank'  units='mult'  use_header_enum=off  row_header_enum={}  col_header_enum={}  use_precision=off  precision=''  gain=1  offset=0  exp=1  use_mototune_group=on  mototune_group=motohawk_vardec_path(gcb)
  motohawk_probe3 : MotoHawk_lib/Calibration & Probing Blocks/motohawk_probe  nam='LiquidO2Control_ErrorTerm_BankA'  show_more=on  name_source=Use Parameter  read_level=1  view_as=Number  enum_struct={'Disabled', 'Enabled'}  vector_style=Wide Row  use_help_units=on  help='Closed-loop O2 control error-term, for bank'  units='mult'  use_header_enum=off  row_header_enum={}  col_header_enum={}  use_precision=off  precision=''  gain=1  offset=0  exp=1  use_mototune_group=on  mototune_group=motohawk_vardec_path(gcb)
  Multiplier : Outport
  ITerm : Outport  Port=2
  wires:
  Reset/1 -> Universal PID/10
  Universal PID/3 -> motohawk_probe/1
  Universal PID/4 -> motohawk_probe1/1, ITerm/1
  Constant/1 -> Universal PID/7
  Universal PID/5 -> motohawk_probe2/1
  Saturation/1 -> Multiplier/1
  O2Sensor/1 -> Universal PID/1
  TargetEquivRatio/1 -> Universal PID/2
  ErrorGain/1 -> Universal PID/3
  PGain/1 -> Universal PID/4
  IGain/1 -> Universal PID/5
  DGain/1 -> Universal PID/6
  OutUpperLimit/1 -> Saturation/3
  Convert to Fuel Multiplier/1 -> Sum/1
  Universal PID/1 -> Sum/2
  Sum/1 -> Saturation/1
  ITermUpperLimit/1 -> Universal PID/9
  ITermLowerLimit/1 -> Universal PID/8
  OutLowerLimit/1 -> Saturation/2
  Universal PID/2 -> motohawk_probe3/1
